simulink model "H_T"  (R2017b)
settings: Solver=VariableStepAuto  StartTime=0.0  StopTime=inf  RelTol=1e-3
libraries: simulink x2, realtime_pacer_lib x1
settings Model: Creator=hattanbadyah  LastModifiedBy=hattanbadyah
settings CodeAppCC: StateflowObjectComments=on

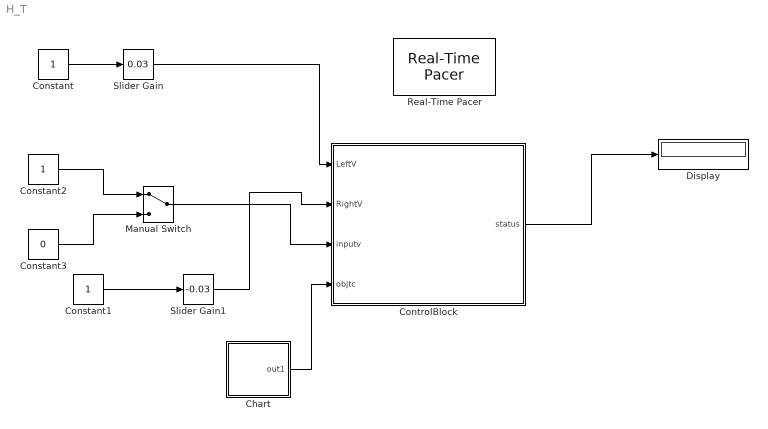
== system H_T ==
  Chart : Stateflow chart  TreatAsAtomicUnit=on
  Constant : Constant
  Constant1 : Constant
  Constant2 : Constant
  Constant3 : Constant  Value=0
  ControlBlock : Stateflow chart  TreatAsAtomicUnit=on
  Display : Display
  Manual Switch : ManualSwitch
  Real-Time Pacer : realtime_pacer_lib/Real-Time Pacer  simTimePerRealTime=1
  Slider Gain : simulink/Math Operations/Slider Gain  gain=0.03  low=-0.5  high=0.5
  Slider Gain1 : simulink/Math Operations/Slider Gain  gain=-0.03  low=-0.5  high=0.5
  wires:
  Constant1/1 -> Slider Gain1/1
  Constant/1 -> Slider Gain/1
  Constant2/1 -> Manual Switch/1
  ControlBlock/1(status) -> Display/1
  Slider Gain/1 -> ControlBlock/1(LeftV)
  Slider Gain1/1 -> ControlBlock/2(RightV)
  Manual Switch/1 -> ControlBlock/3(inputv)
  Constant3/1 -> Manual Switch/2
  Chart/1(out1) -> ControlBlock/4(objtc)

== stateflow chart H_T/Chart ==
  state A
    en,du:
    tcpInit;
    out1 = 1;
  (default) -> A
  data: out1 output
  function tcpInit:
    | function tcpInit
    | coder.extrinsic('tcpip');
    | coder.extrinsic('assignin');
    | persistent obj
    | if isempty(obj)
    |     obj=tcpip('10.0.0.1',9001);
    |     set(obj,'Terminator','LF')
    |     set(obj,'InputBufferSize',1000)
    |     set(obj, 'Timeout', .5)
    |     set(obj, 'ByteOrder','bigEndian');
    |     assignin('base','objWs',obj);
    |     
    | fopen(obj);
    |     % Start!
    | Start=[128];
    | fwrite(obj,Start);
    | pause(.1)
    | Mode=[132]
    | fwrite(obj,Mode);
    | pause(.1)
    | 
    | % %Print 'go' on display
    | fwrite(obj, [164, 71, 79, 32, 32]);
    | % make a sound
    | fwrite(obj, [140 1 3 60 20 72 20 84 40 ]); %RoombaInit Song
    | fwrite(obj, [140 2 1 60 20]); % BeepRoomba song
    | fwrite(obj, [140 3 3 84 20 72 30 60 40]); % PowerOffRoomba song
    | fwrite(obj, [141 1]); % play RoombaInit song
    | disp('Robot should display go on 7 segment LED panel and play song.')
    | pause(1);
    | end

== stateflow chart H_T/ControlBlock ==
  state blank
  state Connect
    entry:
    coder.extrinsic('evalin');
    obj=evalin('base','objWs');
    status= 0
  state Reset_Stop
    entry:
    coder.extrinsic('SetWheelVelRoomba')
    SetWheelVelRoomba(obj,0, 0)
    status=2
  state Update
    entry,during:
    coder.extrinsic('SetWheelVelRoomba')
    SetWheelVelRoomba(obj,RightV, LeftV)
    status=1
  state start
    entry,during:
    coder.extrinsic('SetWheelVelRoomba')
    SetWheelVelRoomba(obj,RightV, LeftV)
    status=1
  (default) -> blank
  blank -> Connect : [objtc==1]
  Reset_Stop -> Connect [order 2] : after(30,sec)
  Connect -> start : [inputv==1]
  Update -> start : after(0.5,sec)
  start -> Reset_Stop [order 1] : [inputv==0]
  Reset_Stop -> start [order 1] : [inputv==1]
  start -> Update [order 2] : after(0.5,sec)
  data: LeftV input; RightV input; inputv input; status output; objtc input; obj local
